simulink model "BCM2_4"  (R2021b)
settings: Solver=FixedStepDiscrete  StartTime=0.0  StopTime=1  FixedStep=0.001  RelTol=1e-3  EnableMultiTasking=on
InitFcn:
  | mbd_mpc_consistency_checks(bdroot(gcs));
model workspace (MAT data in the model file):
  CAN_rec : Simulink.Signal (value not decoded)
  CAN_transm_stat : Simulink.Signal (value not decoded)
  CAN_trm : Simulink.Signal (value not decoded)
  DITHER_CFB0 : Simulink.Parameter (value not decoded)
  DITHER_CFB1 : Simulink.Parameter (value not decoded)
  DITHER_CFB2 : Simulink.Parameter (value not decoded)
  DITHER_EN0 : Simulink.Parameter (value not decoded)
  DITHER_EN1 : Simulink.Parameter (value not decoded)
  DITHER_EN2 : Simulink.Parameter (value not decoded)
  DITHER_SIZE0 : Simulink.Parameter (value not decoded)
  DITHER_SIZE1 : Simulink.Parameter (value not decoded)
  DITHER_SIZE2 : Simulink.Parameter (value not decoded)
  DITHER_STEP0 : Simulink.Parameter (value not decoded)
  DITHER_STEP1 : Simulink.Parameter (value not decoded)
  DITHER_STEP2 : Simulink.Parameter (value not decoded)
  DITHER_SYNC0 : Simulink.Parameter (value not decoded)
  DITHER_SYNC1 : Simulink.Parameter (value not decoded)
  DITHER_SYNC2 : Simulink.Parameter (value not decoded)
  ECUMbut : Simulink.Signal (value not decoded)
  FAULTN : Simulink.Signal (value not decoded)
  FM0 : Simulink.Parameter (value not decoded)
  FM1 : Simulink.Parameter (value not decoded)
  FM2 : Simulink.Parameter (value not decoded)
  FME : Simulink.Parameter (value not decoded)
  Fsys_M : Simulink.Parameter (value not decoded)
  Fsys_N : Simulink.Parameter (value not decoded)
  Fsys_WDEN : Simulink.Parameter (value not decoded)
  Fsys_div : Simulink.Parameter (value not decoded)
  HL0 : Simulink.Parameter (value not decoded)
  HL1 : Simulink.Parameter (value not decoded)
  HL2 : Simulink.Parameter (value not decoded)
  IDIAG0 : Simulink.Parameter (value not decoded)
  IDIAG1 : Simulink.Parameter (value not decoded)
  IDIAG2 : Simulink.Parameter (value not decoded)
  Ivalve : Simulink.Signal (value not decoded)
  KI_index0 : Simulink.Parameter (value not decoded)
  KI_index1 : Simulink.Parameter (value not decoded)
  KI_index2 : Simulink.Parameter (value not decoded)
  PWM_Period0 : Simulink.Parameter (value not decoded)
  PWM_Period1 : Simulink.Parameter (value not decoded)
  PWM_Period2 : Simulink.Parameter (value not decoded)
  RESN : Simulink.Signal (value not decoded)
  SR0 : Simulink.Parameter (value not decoded)
  SR1 : Simulink.Parameter (value not decoded)
  SR2 : Simulink.Parameter (value not decoded)
  Vparam : Simulink.Signal (value not decoded)
  block_tle : Simulink.Signal (value not decoded)
  disp : Simulink.Signal (value not decoded)
  ee_adr : Simulink.Signal (value not decoded)
  ee_en_rd : Simulink.Signal (value not decoded)
  ee_en_wr : Simulink.Signal (value not decoded)
  ee_idle : Simulink.Signal (value not decoded)
  ee_read : Simulink.Signal (value not decoded)
  ee_recv : Simulink.Signal (value not decoded)
  ee_send : Simulink.Signal (value not decoded)
  in_stats : Simulink.Signal (value not decoded)
  inputs : Simulink.Signal (value not decoded)
  light : Simulink.Signal (value not decoded)
  out_drv : Simulink.Signal (value not decoded)
  out_drv_test : Simulink.Signal (value not decoded)
  out_test_en : Simulink.Signal (value not decoded)
  recv_spi2 : Simulink.Signal (value not decoded)
  ret : Simulink.Signal (value not decoded)
  spi_rcv_tle82453 : Simulink.Signal (value not decoded)
  tle82453_Ivlv : Simulink.Signal (value not decoded)
  tle82453_err : Simulink.Signal (value not decoded)
  tle82453_reset : Simulink.Signal (value not decoded)
  wtdg_CAN : Simulink.Signal (value not decoded)
symbols that are objects in the model workspace (value not decoded): CAN_rec, CAN_transm_stat, ECUMbut, inputs, Ivalve, out_drv_test, recv_spi2, ret, SR0, tle82453_Ivlv
undefined symbols (not defined in the file or in its folder): color, LQFP
libraries: simulink x68, mbd_mpc574x_ec_toolbox x50, canmsglib x42, hdlsllib x9, commutil2 x7, etargetslib x4
(part 5 of 6)

== system BCM2_4/CAN_Receive/RX_FIFO_Complete_Event2 buf 22-26/ID0X18FEEA2F buf = 23 ==
  Data : Inport
  Action Port : ActionPort  ActionPortLabel=case [ 419359279 ]:
  Constant : Constant  Value=0  OutDataTypeStr=uint16
  Data Store Write1 : DataStoreWrite  DataStoreName=wtdg_CAN  DataStoreElements=wtdg_CAN.w18FEEA2F  IndexOptions=Index vector (dialog)  Indices=1  OutputSizes=1
  Data Store Write2 : DataStoreWrite  DataStoreName=CAN_rec  DataStoreElements=CAN_rec.m18FEEA2F(:)  IndexOptions=Index vector (dialog)  Indices=1  OutputSizes=1
  wires:
  Constant/1 -> Data Store Write1/1
  Data/1 -> Data Store Write2/1

== system BCM2_4/CAN_Receive/RX_FIFO_Complete_Event2 buf 22-26/ID0X192 buf = 22 ==
  Data : Inport
  Action Port : ActionPort  ActionPortLabel=case [ 402 ]:
  CAN Pack1 : canmsglib/CAN Pack  CANdbFile=C:\Documents\Документация\J1939\j1939.dbc  MsgList=A1  MsgName=CANPACK  MsgIDType=Standard (11-bit identifier)  MsgIdentifier=hex2dec('192')  MsgLength=8  Remote=off  ApplyMinMax=off  BusOutput=off  SignalInfo={}
      settings: SourceProductBaseCode=ME,XP,VN  DataFormat=raw data
  CAN Unpack2 : canmsglib/CAN Unpack  MsgList=(none)  MsgName=Ecu_master_4  MsgIDType=Standard (11-bit identifier)  MsgIdentifier="hex2dec(\"192\")"  MsgLength=8  SignalInfo={ 'Butons', '0', '8', 'LE', 'signed', 'Standard', '0', '1', '0', '-Inf', 'Inf' }  IDPort=off  TimestampPort=off  ErrorPort=off  RemotePort=off  LengthPort=off  StatusPort=off  ApplyMinMax=off
      settings: SourceProductName=Simulink Real-Time
  Constant : Constant  Value=0  OutDataTypeStr=uint16
  Data Store Write : DataStoreWrite  DataStoreName=ECUMbut  DataStoreElements=ECUMbut.arr4(:)  IndexOptions=Index vector (dialog)  Indices=1  OutputSizes=1
  Data Store Write1 : DataStoreWrite  DataStoreName=wtdg_CAN  DataStoreElements=wtdg_CAN.id192  IndexOptions=Index vector (dialog)  Indices=1  OutputSizes=1
  Integer to Bit Converter : commutil2/Integer to Bit Converter  nbits=8  signedInputValues=Unsigned  bitOrder=LSB first  outDtype=boolean
  wires:
  Data/1 -> CAN Pack1/1
  CAN Unpack2/1 -> Integer to Bit Converter/1
  CAN Pack1/1 -> CAN Unpack2/1
  Constant/1 -> Data Store Write1/1
  Integer to Bit Converter/1 -> Data Store Write/1

== system BCM2_4/CAN_Receive/RX_FIFO_Complete_Event2 buf 22-26/ID0X195 buf = 22 ==
  Data : Inport
  Action Port : ActionPort  ActionPortLabel=case [ 405 ]:
  CAN Pack1 : canmsglib/CAN Pack  CANdbFile=C:\Documents\Документация\J1939\j1939.dbc  MsgList=A1  MsgName=CANPACK  MsgIDType=Standard (11-bit identifier)  MsgIdentifier=hex2dec('195')  MsgLength=8  Remote=off  ApplyMinMax=off  BusOutput=off  SignalInfo={}
      settings: SourceProductBaseCode=ME,XP,VN  DataFormat=raw data
  CAN Unpack1 : canmsglib/CAN Unpack  MsgList=(none)  MsgName=ecumaster_12  MsgIDType=Standard (11-bit identifier)  MsgIdentifier="hex2dec(\"195\")"  MsgLength=8  SignalInfo={ 'buttons', '0', '16', 'LE', 'unsigned', 'Standard', '0', '1', '0', '0', 'inf' }  IDPort=off  TimestampPort=off  ErrorPort=off  RemotePort=off  LengthPort=off  StatusPort=off  ApplyMinMax=off
      settings: SourceProductName=Simulink Real-Time
  Constant : Constant  Value=0  OutDataTypeStr=uint16
  Data Store Write : DataStoreWrite  DataStoreName=ECUMbut  DataStoreElements=ECUMbut.arr12(:)  IndexOptions=Index vector (dialog)  Indices=1  OutputSizes=1
  Data Store Write1 : DataStoreWrite  DataStoreName=wtdg_CAN  DataStoreElements=wtdg_CAN.id195  IndexOptions=Index vector (dialog)  Indices=1  OutputSizes=1
  Integer to Bit Converter : commutil2/Integer to Bit Converter  nbits=16  signedInputValues=Unsigned  bitOrder=LSB first  outDtype=boolean
  wires:
  CAN Pack1/1 -> CAN Unpack1/1
  Data/1 -> CAN Pack1/1
  CAN Unpack1/1 -> Integer to Bit Converter/1
  Integer to Bit Converter/1 -> Data Store Write/1
  Constant/1 -> Data Store Write1/1

== system BCM2_4/CAN_Receive/RX_FIFO_Complete_Event2 buf 22-26/reinit buf 22 ==
  Action Port : ActionPort  ActionPortLabel=case [ 22 ]:
  FCAN_Receive_ID_1xx : mbd_mpc574x_ec_toolbox/Communication Blocks/CAN Blocks/FCAN_Receive  can_instance=1  can_mode=Non-blocking  can_timeout_ms=0  can_mb_idx=22  can_extended_id=off  can_is_remote=off  can_id=100  can_msg_mask=FFFFFF00  show_adv_opts=off  can_use_rxfifo=off  can_fd_enable=off
      settings: SourceProductName=NXP Model-Based Design Toolbox for MPC57xx MCUs

== system BCM2_4/CAN_Receive/RX_FIFO_Complete_Event2 buf 22-26/reinit buf 23 ==
  Action Port : ActionPort  ActionPortLabel=case [ 23 ]:
  FCAN_Receive_ID_18Fxxxxx : mbd_mpc574x_ec_toolbox/Communication Blocks/CAN Blocks/FCAN_Receive  can_instance=1  can_mode=Non-blocking  can_timeout_ms=0  can_mb_idx=22  can_extended_id=on  can_is_remote=off  can_id=18F00000  can_msg_mask=FFF00000  show_adv_opts=off  can_use_rxfifo=off  can_fd_enable=off
      settings: SourceProductName=NXP Model-Based Design Toolbox for MPC57xx MCUs

== system BCM2_4/CAN_Receive/RX_FIFO_Complete_Event3 buf 44-48/ID0X192 buf = 15 ==
  Data : Inport
  Action Port : ActionPort
  CAN Pack1 : canmsglib/CAN Pack  CANdbFile=C:\Documents\Документация\J1939\j1939.dbc  MsgList=A1  MsgName=CANPACK  MsgIDType=Standard (11-bit identifier)  MsgIdentifier=hex2dec('192')  MsgLength=8  Remote=off  ApplyMinMax=off  BusOutput=off  SignalInfo={}
      settings: SourceProductBaseCode=ME,XP,VN  DataFormat=raw data
  CAN Unpack2 : canmsglib/CAN Unpack  MsgList=(none)  MsgName=Rear_modulator  MsgIDType=Standard (11-bit identifier)  MsgIdentifier="hex2dec(\"192\")"  MsgLength=8  SignalInfo={ 'Current_pressure', '48', '8', 'LE', 'unsigned', 'Standard', '0', '0.05', '0', '-Inf', 'Inf'; 'Select_pressure', '56', '8', 'LE', 'unsigned', 'Standard', '0', '0.05', '0', '-Inf', 'Inf' }  IDPort=off  TimestampPort=off  ErrorPort=off  RemotePort=off  LengthPort=off  StatusPort=off  ApplyMinMax=off
      settings: SourceProductName=Simulink Real-Time
  Constant : Constant  Value=0  OutDataTypeStr=uint16
  Data Store Write1 : DataStoreWrite  DataStoreName=wtdg_CAN  DataStoreElements=wtdg_CAN.id192  IndexOptions=Index vector (dialog)  Indices=1  OutputSizes=1
  Terminator : Terminator
  Terminator1 : Terminator
  wires:
  Constant/1 -> Data Store Write1/1
  CAN Pack1/1 -> CAN Unpack2/1
  CAN Unpack2/1 -> Terminator/1
  CAN Unpack2/2 -> Terminator1/1
  Data/1 -> CAN Pack1/1

== system BCM2_4/CAN_Receive/RX_FIFO_Complete_Event3 buf 44-48/ID0X195 buf = 15 ==
  Data : Inport
  Action Port : ActionPort
  CAN Pack1 : canmsglib/CAN Pack  CANdbFile=C:\Documents\Документация\J1939\j1939.dbc  MsgList=A1  MsgName=CANPACK  MsgIDType=Standard (11-bit identifier)  MsgIdentifier=hex2dec('195')  MsgLength=8  Remote=off  ApplyMinMax=off  BusOutput=off  SignalInfo={}
      settings: SourceProductBaseCode=ME,XP,VN  DataFormat=raw data
  CAN Unpack1 : canmsglib/CAN Unpack  MsgList=(none)  MsgName=ecumaster_12  MsgIDType=Standard (11-bit identifier)  MsgIdentifier="hex2dec(\"195\")"  MsgLength=8  SignalInfo={ 'buttons', '0', '16', 'LE', 'unsigned', 'Standard', '0', '1', '0', '0', 'inf' }  IDPort=off  TimestampPort=off  ErrorPort=off  RemotePort=off  LengthPort=off  StatusPort=off  ApplyMinMax=off
      settings: SourceProductName=Simulink Real-Time
  Constant : Constant  Value=0  OutDataTypeStr=uint16
  Data Store Write : DataStoreWrite  DataStoreName=ECUMbut  DataStoreElements=ECUMbut.arr12(:)  IndexOptions=Index vector (dialog)  Indices=1  OutputSizes=1
  Data Store Write1 : DataStoreWrite  DataStoreName=wtdg_CAN  DataStoreElements=wtdg_CAN.id195  IndexOptions=Index vector (dialog)  Indices=1  OutputSizes=1
  Integer to Bit Converter : commutil2/Integer to Bit Converter  nbits=16  signedInputValues=Unsigned  bitOrder=LSB first  outDtype=boolean
  wires:
  Constant/1 -> Data Store Write1/1
  Integer to Bit Converter/1 -> Data Store Write/1
  CAN Unpack1/1 -> Integer to Bit Converter/1
  Data/1 -> CAN Pack1/1
  CAN Pack1/1 -> CAN Unpack1/1

== system BCM2_4/CAN_Receive/RX_FIFO_Complete_Event3 buf 44-48/reinit buf 15 ==
  Action Port : ActionPort
  FCAN_Receive_ID_1xx : mbd_mpc574x_ec_toolbox/Communication Blocks/CAN Blocks/FCAN_Receive  can_instance=1  can_mode=Non-blocking  can_timeout_ms=0  can_mb_idx=15  can_extended_id=off  can_is_remote=off  can_id=100  can_msg_mask=FFFFFF00  show_adv_opts=off  can_use_rxfifo=off  can_fd_enable=off
      settings: SourceProductName=NXP Model-Based Design Toolbox for MPC57xx MCUs

== system BCM2_4/Drivers/Diagnostic1/Switch Case Action Subsystem ==
  In1 : Inport
  Action Port : ActionPort  ActionPortLabel=case [ 2 ]:
  Byte Unpack1 : etargetslib/Byte Unpack  dimensions={[1]}  datatypes={'uint32'}  byteAlign=4
  Constant : Constant  Value=0  OutDataTypeStr=uint8  SampleTime=-1
  Data Store Write : DataStoreWrite  DataStoreName=tle82453_err  IndexOptions=Index vector (dialog)  Indices=1  OutputSizes=1
  Mux : Mux  Inputs=2
  wires:
  Byte Unpack1/1 -> Data Store Write/1
  In1/1 -> Mux/2
  Mux/1 -> Byte Unpack1/1
  Constant/1 -> Mux/1

== system BCM2_4/Drivers/Diagnostic1/Switch Case Action Subsystem1 ==
  In1 : Inport
  Action Port : ActionPort  ActionPortLabel=case [ 64 ]:
  Add : Sum  Inputs=3
  Bit Shift1 : hdlsllib/Logic and Bit Operations/Bit Shift  mode=Shift Left Logical  N=8
  Bit Shift2 : hdlsllib/Logic and Bit Operations/Bit Shift  mode=Shift Right Logical  N=12
  Bit Shift3 : hdlsllib/Logic and Bit Operations/Bit Shift  mode=Shift Left Logical  N=16
  Bitwise AND : simulink/Logic and Bit Operations/Bitwise Operator  logicop=AND  UseBitMask=on  BitMask=bin2dec('000000000000111111111111')  BitMaskRealWorld=Stored Integer
  Data Store Write1 : DataStoreWrite  DataStoreName=tle82453_Ivlv  DataStoreElements=tle82453_Ivlv(1)  IndexOptions=Index vector (dialog)  Indices=1  OutputSizes=1
  Data Type Conversion : DataTypeConversion  OutDataTypeStr=uint32
  Data Type Conversion1 : DataTypeConversion  OutDataTypeStr=double
  Data Type Conversion2 : DataTypeConversion  OutDataTypeStr=double
  Data Type Conversion3 : DataTypeConversion  OutDataTypeStr=uint8
  Demux : Demux  Outputs=3
  Gain : Gain  Gain=150  OutDataTypeStr=double
  Multiply : Product  Inputs=*/  OutDataTypeStr=double
  wires:
  Bitwise AND/1 -> Data Type Conversion2/1
  Data Type Conversion2/1 -> Multiply/2
  Gain/1 -> Multiply/1
  Add/1 -> Bitwise AND/1, Bit Shift2/1
  Bit Shift3/1 -> Add/1
  Demux/3 -> Add/3
  Bit Shift2/1 -> Data Type Conversion1/1
  Data Type Conversion1/1 -> Gain/1
  Demux/1 -> Bit Shift3/1
  Bit Shift1/1 -> Add/2
  Demux/2 -> Bit Shift1/1
  Data Type Conversion/1 -> Demux/1
  In1/1 -> Data Type Conversion/1
  Data Type Conversion3/1 -> Data Store Write1/1
  Multiply/1 -> Data Type Conversion3/1

== system BCM2_4/Drivers/Diagnostic1/Switch Case Action Subsystem2 ==
  In1 : Inport
  Action Port : ActionPort  ActionPortLabel=case [ 65 ]:
  Add : Sum  Inputs=3
  Bit Shift1 : hdlsllib/Logic and Bit Operations/Bit Shift  mode=Shift Left Logical  N=8
  Bit Shift2 : hdlsllib/Logic and Bit Operations/Bit Shift  mode=Shift Right Logical  N=12
  Bit Shift3 : hdlsllib/Logic and Bit Operations/Bit Shift  mode=Shift Left Logical  N=16
  Bitwise AND : simulink/Logic and Bit Operations/Bitwise Operator  logicop=AND  UseBitMask=on  BitMask=bin2dec('000000000000111111111111')  BitMaskRealWorld=Stored Integer
  Data Store Write2 : DataStoreWrite  DataStoreName=tle82453_Ivlv  DataStoreElements=tle82453_Ivlv(2)  IndexOptions=Index vector (dialog)  Indices=1  OutputSizes=1
  Data Type Conversion : DataTypeConversion  OutDataTypeStr=uint32
  Data Type Conversion1 : DataTypeConversion  OutDataTypeStr=double
  Data Type Conversion2 : DataTypeConversion  OutDataTypeStr=double
  Data Type Conversion3 : DataTypeConversion  OutDataTypeStr=uint8
  Demux : Demux  Outputs=3
  Gain : Gain  Gain=150  OutDataTypeStr=double
  Multiply : Product  Inputs=*/  OutDataTypeStr=double
  wires:
  Bit Shift2/1 -> Data Type Conversion1/1
  Demux/2 -> Bit Shift1/1
  Data Type Conversion/1 -> Demux/1
  Bit Shift1/1 -> Add/2
  Demux/3 -> Add/3
  Add/1 -> Bitwise AND/1, Bit Shift2/1
  Bit Shift3/1 -> Add/1
  Demux/1 -> Bit Shift3/1
  In1/1 -> Data Type Conversion/1
  Bitwise AND/1 -> Data Type Conversion2/1
  Gain/1 -> Multiply/1
  Data Type Conversion1/1 -> Gain/1
  Data Type Conversion2/1 -> Multiply/2
  Data Type Conversion3/1 -> Data Store Write2/1
  Multiply/1 -> Data Type Conversion3/1

== system BCM2_4/Drivers/Diagnostic1/Switch Case Action Subsystem3 ==
  In1 : Inport
  Action Port : ActionPort  ActionPortLabel=case [ 66 ]:
  Add : Sum  Inputs=3
  Bit Shift1 : hdlsllib/Logic and Bit Operations/Bit Shift  mode=Shift Left Logical  N=8
  Bit Shift2 : hdlsllib/Logic and Bit Operations/Bit Shift  mode=Shift Right Logical  N=12
  Bit Shift3 : hdlsllib/Logic and Bit Operations/Bit Shift  mode=Shift Left Logical  N=16
  Bitwise AND : simulink/Logic and Bit Operations/Bitwise Operator  logicop=AND  UseBitMask=on  BitMask=bin2dec('000000000000111111111111')  BitMaskRealWorld=Stored Integer
  Data Store Write3 : DataStoreWrite  DataStoreName=tle82453_Ivlv  DataStoreElements=tle82453_Ivlv(3)  IndexOptions=Index vector (dialog)  Indices=1  OutputSizes=1
  Data Type Conversion : DataTypeConversion  OutDataTypeStr=uint32
  Data Type Conversion1 : DataTypeConversion  OutDataTypeStr=double
  Data Type Conversion2 : DataTypeConversion  OutDataTypeStr=double
  Data Type Conversion3 : DataTypeConversion  OutDataTypeStr=uint8
  Demux : Demux  Outputs=3
  Gain : Gain  Gain=150  OutDataTypeStr=double
  Multiply : Product  Inputs=*/  OutDataTypeStr=double
  wires:
  In1/1 -> Data Type Conversion/1
  Bitwise AND/1 -> Data Type Conversion2/1
  Data Type Conversion2/1 -> Multiply/2
  Gain/1 -> Multiply/1
  Add/1 -> Bitwise AND/1, Bit Shift2/1
  Bit Shift3/1 -> Add/1
  Demux/3 -> Add/3
  Bit Shift2/1 -> Data Type Conversion1/1
  Data Type Conversion1/1 -> Gain/1
  Demux/1 -> Bit Shift3/1
  Bit Shift1/1 -> Add/2
  Demux/2 -> Bit Shift1/1
  Data Type Conversion/1 -> Demux/1
  Data Type Conversion3/1 -> Data Store Write3/1
  Multiply/1 -> Data Type Conversion3/1

== system BCM2_4/Drivers/input status/Switch Case Action Subsystem ==
  Action Port : ActionPort  ActionPortLabel=case [ 62 ]:
  Byte Unpack : etargetslib/Byte Unpack  dimensions={[1]}  datatypes={'uint32'}  byteAlign=4
  Data Store Read1 : DataStoreRead  DataStoreName=recv_spi2  DataStoreElements=recv_spi2(1:4)  IndexOptions=Index vector (dialog)  Indices=1  OutputSizes=1
  Data Store Write1 : DataStoreWrite  DataStoreName=inputs  DataStoreElements=inputs(1:22)  IndexOptions=Index vector (dialog)  Indices=1  OutputSizes=1
  Integer to Bit Converter1 : commutil2/Integer to Bit Converter  nbits=32  signedInputValues=Unsigned  bitOrder=LSB first  outDtype=boolean
  Selector2 : Selector  InputPortWidth=32  IndexOptions=Index vector (dialog)  Indices=[1:22]  OutputSizes=1
  wires:
  Selector2/1 -> Data Store Write1/1
  Integer to Bit Converter1/1 -> Selector2/1
  Data Store Read1/1 -> Byte Unpack/1
  Byte Unpack/1 -> Integer to Bit Converter1/1

== system BCM2_4/Drivers/input status/Switch Case Action Subsystem1 ==
  Action Port : ActionPort  ActionPortLabel=default:

== system BCM2_4/Drivers/input status/Switch Case Action Subsystem2 ==
  Action Port : ActionPort  ActionPortLabel=case [ 62 ]:
  Byte Unpack : etargetslib/Byte Unpack  dimensions={[1]}  datatypes={'uint32'}  byteAlign=4
  Data Store Read : DataStoreRead  DataStoreName=recv_spi2  DataStoreElements=recv_spi2(5:8)  IndexOptions=Index vector (dialog)  Indices=1  OutputSizes=1
  Data Store Write : DataStoreWrite  DataStoreName=inputs  DataStoreElements=inputs(23:44)  IndexOptions=Index vector (dialog)  Indices=1  OutputSizes=1
  Integer to Bit Converter1 : commutil2/Integer to Bit Converter  nbits=32  signedInputValues=Unsigned  bitOrder=LSB first  outDtype=boolean
  Selector2 : Selector  InputPortWidth=32  IndexOptions=Index vector (dialog)  Indices=[1:22]  OutputSizes=1
  wires:
  Byte Unpack/1 -> Integer to Bit Converter1/1
  Selector2/1 -> Data Store Write/1
  Integer to Bit Converter1/1 -> Selector2/1
  Data Store Read/1 -> Byte Unpack/1

== system BCM2_4/Drivers/input status/Switch Case Action Subsystem3 ==
  Action Port : ActionPort  ActionPortLabel=default:

== system BCM2_4/Init System/Начальная иницилизация/Init filters CAN ==
  FCAN_Receive_ID_0CFxxxxx : mbd_mpc574x_ec_toolbox/Communication Blocks/CAN Blocks/FCAN_Receive  can_instance=0  can_mode=Non-blocking  can_timeout_ms=0  can_mb_idx=0  can_extended_id=on  can_is_remote=off  can_id=0CF00000  can_msg_mask=FFF00000  show_adv_opts=off  can_use_rxfifo=off  can_fd_enable=off
      settings: SourceProductName=NXP Model-Based Design Toolbox for MPC57xx MCUs
  FCAN_Receive_ID_1811xxxxx : mbd_mpc574x_ec_toolbox/Communication Blocks/CAN Blocks/FCAN_Receive  can_instance=0  can_mode=Non-blocking  can_timeout_ms=0  can_mb_idx=2  can_extended_id=on  can_is_remote=off  can_id=18110000  can_msg_mask=FFFF0000  show_adv_opts=off  can_use_rxfifo=off  can_fd_enable=off
      settings: SourceProductName=NXP Model-Based Design Toolbox for MPC57xx MCUs
  FCAN_Receive_ID_18Fxxxxx : mbd_mpc574x_ec_toolbox/Communication Blocks/CAN Blocks/FCAN_Receive  can_instance=0  can_mode=Non-blocking  can_timeout_ms=0  can_mb_idx=1  can_extended_id=on  can_is_remote=off  can_id=18F00000  can_msg_mask=FFF00000  show_adv_opts=off  can_use_rxfifo=off  can_fd_enable=off
      settings: SourceProductName=NXP Model-Based Design Toolbox for MPC57xx MCUs
  FCAN_Receive_ID_18Fxxxxx1 : mbd_mpc574x_ec_toolbox/Communication Blocks/CAN Blocks/FCAN_Receive  can_instance=1  can_mode=Non-blocking  can_timeout_ms=0  can_mb_idx=22  can_extended_id=on  can_is_remote=off  can_id=18F00000  can_msg_mask=FFF00000  show_adv_opts=off  can_use_rxfifo=off  can_fd_enable=off
      settings: SourceProductName=NXP Model-Based Design Toolbox for MPC57xx MCUs
  FCAN_Receive_ID_1FEEF888 : mbd_mpc574x_ec_toolbox/Communication Blocks/CAN Blocks/FCAN_Receive  can_instance=0  can_mode=Non-blocking  can_timeout_ms=0  can_mb_idx=3  can_extended_id=on  can_is_remote=off  can_id=1FEEF888  can_msg_mask=FFFFFFFF  show_adv_opts=off  can_use_rxfifo=off  can_fd_enable=off
      settings: SourceProductName=NXP Model-Based Design Toolbox for MPC57xx MCUs
  FCAN_Receive_ID_1xx : mbd_mpc574x_ec_toolbox/Communication Blocks/CAN Blocks/FCAN_Receive  can_instance=1  can_mode=Non-blocking  can_timeout_ms=0  can_mb_idx=22  can_extended_id=off  can_is_remote=off  can_id=100  can_msg_mask=FFFFFF00  show_adv_opts=off  can_use_rxfifo=off  can_fd_enable=off
      settings: SourceProductName=NXP Model-Based Design Toolbox for MPC57xx MCUs

== system BCM2_4/Степы ретардера/страницы механика+/Subsystem ==
  Enable : EnablePort
  Add : Sum
  Constant : Constant  OutDataTypeStr=uint8
  Data Store Read : DataStoreRead  DataStoreName=ret  DataStoreElements=ret.step  IndexOptions=Index vector (dialog)  Indices=1  OutputSizes=1
  Data Store Write : DataStoreWrite  DataStoreName=ret  DataStoreElements=ret.step  IndexOptions=Index vector (dialog)  Indices=1  OutputSizes=1
  wires:
  Constant/1 -> Add/2
  Data Store Read/1 -> Add/1
  Add/1 -> Data Store Write/1

== system BCM2_4/Степы ретардера/страницы механика+/Subsystem1 ==
  Enable : EnablePort
  Add : Sum
  Constant : Constant  OutDataTypeStr=uint8
  Data Store Read : DataStoreRead  DataStoreName=ret  DataStoreElements=ret.step_brk  IndexOptions=Index vector (dialog)  Indices=1  OutputSizes=1
  Data Store Write : DataStoreWrite  DataStoreName=ret  DataStoreElements=ret.step_brk  IndexOptions=Index vector (dialog)  Indices=1  OutputSizes=1
  wires:
  Add/1 -> Data Store Write/1
  Data Store Read/1 -> Add/1
  Constant/1 -> Add/2

== system BCM2_4/Степы ретардера/страницы механика-/Subsystem ==
  Enable : EnablePort
  Add : Sum  Inputs=+-
  Constant : Constant  OutDataTypeStr=uint8
  Data Store Read : DataStoreRead  DataStoreName=ret  DataStoreElements=ret.step  IndexOptions=Index vector (dialog)  Indices=1  OutputSizes=1
  Data Store Write : DataStoreWrite  DataStoreName=ret  DataStoreElements=ret.step  IndexOptions=Index vector (dialog)  Indices=1  OutputSizes=1
  wires:
  Add/1 -> Data Store Write/1
  Data Store Read/1 -> Add/1
  Constant/1 -> Add/2

== system BCM2_4/Топливные баки/Enabled Subsystem/Subsystem ==
  Enable : EnablePort
  Add : Sum  Inputs=+-
  Add1 : Sum
  Constant : Constant  Value=0.8
  Constant1 : Constant  Value=0.8
  Data Store Read : DataStoreRead  DataStoreName=tank1  SampleTime=1  IndexOptions=Index vector (dialog)  Indices=1  OutputSizes=1
  Data Store Read1 : DataStoreRead  DataStoreName=tank3  SampleTime=1  IndexOptions=Index vector (dialog)  Indices=1  OutputSizes=1
  Data Store Write : DataStoreWrite  DataStoreName=tank1  IndexOptions=Index vector (dialog)  Indices=1  OutputSizes=1
  Data Store Write1 : DataStoreWrite  DataStoreName=tank3  IndexOptions=Index vector (dialog)  Indices=1  OutputSizes=1
  wires:
  Constant/1 -> Add/2
  Add/1 -> Data Store Write/1
  Data Store Read/1 -> Add/1
  Data Store Read1/1 -> Add1/1
  Add1/1 -> Data Store Write1/1
  Constant1/1 -> Add1/2

== system BCM2_4/Топливные баки/Enabled Subsystem1/Subsystem ==
  Enable : EnablePort
  Add : Sum  Inputs=+-
  Add1 : Sum
  Constant : Constant  Value=0.8
  Constant1 : Constant  Value=0.8
  Data Store Read : DataStoreRead  DataStoreName=tank2  SampleTime=1  IndexOptions=Index vector (dialog)  Indices=1  OutputSizes=1
  Data Store Read1 : DataStoreRead  DataStoreName=tank3  SampleTime=1  IndexOptions=Index vector (dialog)  Indices=1  OutputSizes=1
  Data Store Write : DataStoreWrite  DataStoreName=tank2  IndexOptions=Index vector (dialog)  Indices=1  OutputSizes=1
  Data Store Write1 : DataStoreWrite  DataStoreName=tank3  IndexOptions=Index vector (dialog)  Indices=1  OutputSizes=1
  wires:
  Constant1/1 -> Add1/2
  Add1/1 -> Data Store Write1/1
  Data Store Read1/1 -> Add1/1
  Data Store Read/1 -> Add/1
  Add/1 -> Data Store Write/1
  Constant/1 -> Add/2

== system BCM2_4/Управление с клавиатуры ECUMASTER/Переключение таблиц ДВС/сброс на ноль ==
  Enable : EnablePort
  Constant : Constant  Value=0  OutDataTypeStr=uint8
  Data Store Write1 : DataStoreWrite  DataStoreName=ECUMbut  DataStoreElements=ECUMbut.cnt(2)  IndexOptions=Index vector (dialog)  Indices=1  OutputSizes=1
  wires:
  Constant/1 -> Data Store Write1/1

== system BCM2_4/Управление с клавиатуры ECUMASTER/Управление габаритами и ближним2/сброс на ноль ==
  Enable : EnablePort
  Constant : Constant  Value=0  OutDataTypeStr=uint8
  Data Store Write1 : DataStoreWrite  DataStoreName=ECUMbut  DataStoreElements=ECUMbut.cnt(1)  IndexOptions=Index vector (dialog)  Indices=1  OutputSizes=1
  wires:
  Constant/1 -> Data Store Write1/1

== system BCM2_4/управление страницами и яркостью мониторов/страницы механика+/Subsystem ==
  Enable : EnablePort
  Add : Sum
  Constant : Constant  OutDataTypeStr=uint8
  Data Store Read : DataStoreRead  DataStoreName=disp  DataStoreElements=disp.meh_page  IndexOptions=Index vector (dialog)  Indices=1  OutputSizes=1
  Data Store Write : DataStoreWrite  DataStoreName=disp  DataStoreElements=disp.meh_page  IndexOptions=Index vector (dialog)  Indices=1  OutputSizes=1
  wires:
  Constant/1 -> Add/2
  Data Store Read/1 -> Add/1
  Add/1 -> Data Store Write/1

== system BCM2_4/управление страницами и яркостью мониторов/страницы механика-/Subsystem ==
  Enable : EnablePort
  Add : Sum  Inputs=+-
  Constant : Constant  OutDataTypeStr=uint8
  Data Store Read : DataStoreRead  DataStoreName=disp  DataStoreElements=disp.meh_page  IndexOptions=Index vector (dialog)  Indices=1  OutputSizes=1
  Data Store Write : DataStoreWrite  DataStoreName=disp  DataStoreElements=disp.meh_page  IndexOptions=Index vector (dialog)  Indices=1  OutputSizes=1
  wires:
  Add/1 -> Data Store Write/1
  Data Store Read/1 -> Add/1
  Constant/1 -> Add/2

== system BCM2_4/управление страницами и яркостью мониторов/страницы пилота+/Subsystem ==
  Enable : EnablePort
  Add : Sum
  Constant : Constant  OutDataTypeStr=uint8
  Data Store Read : DataStoreRead  DataStoreName=disp  DataStoreElements=disp.pilot_page  IndexOptions=Index vector (dialog)  Indices=1  OutputSizes=1
  Data Store Write : DataStoreWrite  DataStoreName=disp  DataStoreElements=disp.pilot_page  IndexOptions=Index vector (dialog)  Indices=1  OutputSizes=1
  wires:
  Add/1 -> Data Store Write/1
  Data Store Read/1 -> Add/1
  Constant/1 -> Add/2

== system BCM2_4/управление страницами и яркостью мониторов/страницы пилота-/Subsystem ==
  Enable : EnablePort
  Add : Sum  Inputs=+-
  Constant : Constant  OutDataTypeStr=uint8
  Data Store Read : DataStoreRead  DataStoreName=disp  DataStoreElements=disp.pilot_page  IndexOptions=Index vector (dialog)  Indices=1  OutputSizes=1
  Data Store Write : DataStoreWrite  DataStoreName=disp  DataStoreElements=disp.pilot_page  IndexOptions=Index vector (dialog)  Indices=1  OutputSizes=1
  wires:
  Constant/1 -> Add/2
  Data Store Read/1 -> Add/1
  Add/1 -> Data Store Write/1

== stateflow chart BCM2_4/Drivers/Driver TLE82453-3 ==
  settings: updateMethod=DISCRETE  sampleTime=0.001
  state Start
    state Init_Vars1
      CLK_DIVIDER = 0x83000000
      CLK_DIVIDER =bitor(CLK_DIVIDER , bitshift(Fsys_WDEN, 12))
      CLK_DIVIDER =bitor(CLK_DIVIDER , bitshift(Fsys_M, 6))
      CLK_DIVIDER =bitor(CLK_DIVIDER , bitshift(Fsys_N, 2))
      CLK_DIVIDER =bitor(CLK_DIVIDER , Fsys_div)
      %-------------------------------------------------------------------------------------
      PWM_PERIOD0 = 0xA8000000
      PWM_PERIOD0 =bitor(PWM_PERIOD0 , bitshift(0, 24))
      PWM_PERIOD0 =bitor(PWM_PERIOD0 , bitshift(KI_index0, 20))
      PWM_PERIOD0 =bitor(PWM_PERIOD0 , PWM_Period0)
      PWM_PERIOD1 = 0xA8000000
      PWM_PERIOD1 =bitor(PWM_PERIOD1 , bitshift(1, 24))
      PWM_PERIOD1 =bitor(PWM_PERIOD1 , bitshift(KI_index1, 20))
      PWM_PERIOD1 =bitor(PWM_PERIOD1 , PWM_Period1)
      PWM_PERIOD2 = 0xA8000000
      PWM_PERIOD2 =bitor(PWM_PERIOD2 , bitshift(2, 24))
      PWM_PERIOD2 =bitor(PWM_PERIOD2 , bitshift(KI_index2, 20))
      PWM_PERIOD2 =bitor(PWM_PERIOD2 , PWM_Period2)
      %--------------------------------------------------------------------------------------
      DITHER0 = 0x98000000
      DITHER0 =bitor(DITHER0 , bitshift(0, 24))
      DITHER0 =bitor(DITHER0 , bitshift(DITHER_EN0, 23))
      DITHER0 =bitor(DITHER0 , bitshift(DITHER_SYNC0, 22))
      DITHER0 =bitor(DITHER0 , bitshift(DITHER_CFB0, 21))
      DITHER0 =bitor(DITHER0 , bitshift(DITHER_STEP0, 10))
      DITHER0 =bitor(DITHER0 , DITHER_SIZE0)
      DITHER1 = 0x98000000
      DITHER1 =bitor(DITHER1 , bitshift(1, 24))
      DITHER1 =bitor(DITHER1 , bitshift(DITHER_EN1, 23))
      DITHER1 =bitor(DITHER1 , bitshift(DITHER_SYNC1, 22))
      DITHER1 =bitor(DITHER1 , bitshift(DITHER_CFB1, 21))
      DITHER1 =bitor(DITHER1 , bitshift(DITHER_STEP1, 10))
      DITHER1 =bitor(DITHER1 , DITHER_SIZE1)
      DITHER2 = 0x98000000
      DITHER2 =bitor(DITHER2 , bitshift(1, 24))
      DITHER2 =bitor(DITHER2 , bitshift(DITHER_EN2, 23))
      DITHER2 =bitor(DITHER2 , bitshift(DITHER_SYNC2, 22))
      DITHER2 =bitor(DITHER2 , bitshift(DITHER_CFB2, 21))
      DITHER2 =bitor(DITHER2 , bitshift(DITHER_STEP2, 10))
      DITHER2 =bitor(DITHER2 , DITHER_SIZE2)
      %-------------------------------------------------------------------------------------
      CONF_REGISTER = 0x81000000
      CONF_REGISTER =bitor(CONF_REGISTER , bitshift((IDIAG2 - 1), 15))
      CONF_REGISTER =bitor(CONF_REGISTER , bitshift((IDIAG1 - 1), 14))
      CONF_REGISTER =bitor(CONF_REGISTER , bitshift((IDIAG0 - 1), 13))
      CONF_REGISTER =bitor(CONF_REGISTER , bitshift((SR2 - 1), 11))
      CONF_REGISTER =bitor(CONF_REGISTER , bitshift((SR1 - 1), 9))
      CONF_REGISTER =bitor(CONF_REGISTER , bitshift((SR0 - 1), 7))
      CONF_REGISTER =bitor(CONF_REGISTER , bitshift((FME - 1), 6))
      CONF_REGISTER =bitor(CONF_REGISTER , bitshift((FM2 - 1), 5))
      CONF_REGISTER =bitor(CONF_REGISTER , bitshift((FM1 - 1), 4))
      CONF_REGISTER =bitor(CONF_REGISTER , bitshift((FM0 - 1), 3))
      CONF_REGISTER =bitor(CONF_REGISTER , bitshift((HL2 - 1), 2))
      CONF_REGISTER =bitor(CONF_REGISTER , bitshift((HL1 - 1), 1))
      CONF_REGISTER =bitor(CONF_REGISTER , (HL0 - 1))
      %init_reg = typecast(swapbytes(CLK_DIVIDER), 'uint8')
      init_reg = typecast(CLK_DIVIDER, 'uint8')
      pwm_reg0 = typecast(PWM_PERIOD0, 'uint8')
      pwm_reg1 = typecast(PWM_PERIOD1, 'uint8')
      pwm_reg2 = typecast(PWM_PERIOD2, 'uint8')
      dith_reg0 = typecast(DITHER0, 'uint8')
      dith_reg1 = typecast(DITHER1, 'uint8')
      dith_reg2 = typecast(DITHER2, 'uint8')
      conf_reg = typecast(CONF_REGISTER, 'uint8')
    state init1
      RESN = false
    state init
      RESN = true
    state out_data
      out = init_reg
      send_spi
    state send
      out2 =  [0X30, bitand(out_drv,255,'uint16')]
      send_spi2
    state send1
      out2 = [0X3F, bitshift(out_drv,-8)]
      send_spi2
    (default) -> Init_Vars1
    Init_Vars1 -> init1
    init1 -> init
    init -> out_data
    send1 -> out_data
    out_data -> send
    send -> send1
  state Work_cycle
    state Setpoint
      out=SP
      res=setpoint(ch+1)*1.364
      IH_temp = bitshift(res,-8,'uint16')
      IL_temp = bitand(res,255,'uint16')
      out(1)=bitor(SP(1), ch)
      out(3)=IH_temp
      out(4)=IL_temp
      ch=ch+1
      send_spi
    state Feedback
      out=FB
      out(1)=bitor(FB(1), ch)
      ch=ch+1
      send_spi
    state Diag
      out=DIAG
      send_spi
    state send2
      out2 = [0X30, bitand(out_drv,255,'uint16')]
      send_spi2
    state send3
      out2 = [0X3F, bitshift(out_drv,-8)]
      send_spi2
    (default) -> Setpoint
    send3 -> Setpoint
    Setpoint -> Feedback : [ch>2]{ch=0}
    Feedback -> Diag : [ch>2]{ch=0}
    Diag -> send2
    send2 -> send3
  state CONFIG1
    state Autozero
      out=Autozero
      out(1) = bitor(Autozero(1),ch)
      ch = ch +1
      send_spi
    state Config
      out=conf_reg;
      send_spi
    state THRESHOLD
      out=ITO
      out(1) = bitor(ITO(1),ch)
      ch=ch+1
      send_spi
    state LIMIT
      out=IL
      out(1) = bitor(IL(1),ch)
      ch=ch+1
      send_spi
    (default) -> Autozero
    Autozero -> Config : [ch>2]{ch=0}
    Config -> THRESHOLD
    THRESHOLD -> LIMIT : [ch>2]{ch=0}
  state PWM_period1
    out=pwm_reg0
    send_spi
  state PWM_period2
    out=pwm_reg1
    send_spi
  state PWM_period3
    out=pwm_reg2
    send_spi
  state Dither1
    out=dith_reg0
    send_spi
  state Dither2
    out=dith_reg1
    send_spi
  state Dither3
    out=dith_reg2
    send_spi
  (default) -> Start
  Work_cycle -> Start : [FAULTN==false || RESET >0]
  Start -> CONFIG1 : [FAULTN==true]{ch=0;}
  CONFIG1 -> Start [order 1] : [FAULTN==false || RESET >0]
  CONFIG1 -> PWM_period1 [order 2] : [ch>2]{ch=0}
  PWM_period1 -> PWM_period2
  PWM_period2 -> PWM_period3
  Dither3 -> Work_cycle
  PWM_period3 -> Dither1
  Dither1 -> Dither2
  Dither2 -> Dither3
  data: Fsys_div parameter uint32 size=1; Fsys_N parameter uint32 size=1; Fsys_M parameter uint32 size=1; Fsys_WDEN parameter uint32 size=1; PWM_Period1 parameter uint32 size=1; PWM_Period2 parameter uint32 size=1; KI_index0 parameter uint32 size=1; KI_index1 parameter uint32 size=1; KI_index2 parameter uint32 size=1; PWM_PERIOD1 local uint32 size=1; PWM_PERIOD2 local uint32 size=1; PWM_Period0 parameter uint32 size=1; PWM_PERIOD0 local uint32 size=1; DITHER_EN0 parameter uint32 size=1; DITHER_EN1 parameter uint32 size=1; DITHER_EN2 parameter uint32 size=1; DITHER_SYNC0 parameter uint32 size=1; DITHER_SYNC1 parameter uint32 size=1; DITHER_SYNC2 parameter uint32 size=1; DITHER_CFB0 parameter uint32 size=1; DITHER_CFB1 parameter uint32 size=1; DITHER_CFB2 parameter uint32 size=1; DITHER_STEP0 parameter uint32 size=1; DITHER_STEP1 parameter uint32 size=1; DITHER_STEP2 parameter uint32 size=1; DITHER_SIZE0 parameter uint32 size=1; DITHER_SIZE1 parameter uint32 size=1; DITHER_SIZE2 parameter uint32 size=1; DITHER1 local uint32 size=1; DITHER2 local uint32 size=1; CLK_DIVIDER local uint32 size=1; ITO local uint8 size=[1 4] =[0XB0 0X00 0X00 0X00]; Autozero constant uint8 size=[1 4] =[0XB8 0X80 0X00 0X00]; SP local uint8 size=[1 4] =[0X90 0XC0 0X00 0X00]; FB local uint8 size=[1 4] =[0X40 0X00 0X00 0X00]; DIAG local uint8 size=[1 4] =[0X02 0X00 0X00 0X00]; IL local uint8 size=[1 4] =[0XA0 0XC8 0X0C 0X80]; IDIAG0 parameter uint32 size=1; CONF_REGISTER local uint32 size=1; SR0 parameter uint32 size=1; FME parameter uint32 size=1; FM0 parameter uint32 size=1; HL0 parameter uint32 size=1; SR1 parameter uint32 size=1; SR2 parameter uint32 size=1; FM1 parameter uint32 size=1; FM2 parameter uint32 size=1; IDIAG1 parameter uint32 size=1; IDIAG2 parameter uint32 size=1; HL1 parameter uint32 size=1; HL2 parameter uint32 size=1; DITHER0 local uint32 size=1; init_reg local uint8 size=[1 4]; pwm_reg0 local uint8 size=[1 4]; dith_reg0 local uint8 size=[1 4]; conf_reg local uint8 size=[1 4]; pwm_reg1 local uint8 size=[1 4]; pwm_reg2 local uint8 size=[1 4]; dith_reg1 local uint8 size=[1 4]; dith_reg2 local uint8 size=[1 4]; ch local uint8 size=1; FAULTN input boolean; RESET input boolean size=1; RESN output boolean size=1; setpoint input uint16 size=[1 3]; IH_temp local; IL_temp local; res local; out output uint8 size=[1 4]; out2 output uint8 size=[1 2]; out_drv input uint16 size=1
  events: send_spi output FUNCTION_CALL_EVENT; send_spi2 output FUNCTION_CALL_EVENT

== stateflow chart BCM2_4/CAN1 Transmit buf 27-43/Цвет клавиатуры 4 buf = 30/Цвет клавиатуры buf = 30/Chart ==
  (default) -> (junction 58)
  (junction 58) -> (junction 46) : {temp=0;}
  (junction 46) -> (junction 48) : {i=0;}
  (junction 48) -> (junction 57) [order 2] : {out[0] = (temp & 255);
      |  out[1] = (temp>>8) & 255;
      |  out[2] = (temp>>16)  & 255;
      |  out[3] = (temp>>24)  & 255;}
  (junction 48) -> (junction 47) [order 1] : [i<4]
  (junction 50) -> (junction 48)
  (junction 47) -> (junction 49) : {temp = temp | (input[i] & 1) << (0+i);
      | temp = temp | ((input[i] & 2)>>1) << (8 + i);
      | temp = temp | ((input[i] & 4)>>2) << (16 + i);}
  (junction 49) -> (junction 50) : {i++;}
  data: i local uint8 size=1 =uint8(0); input input uint8 size=4; temp local double size=1; out output uint8 size=8

== stateflow chart BCM2_4/Drivers/EEPROM DRIVER1 ==
  state start
  state Delay4
  state read_ee
    temp_adress = uint16(adress*2)
    hi_temp = bitshift(temp_adress,-8,'uint16')
    low_temp = bitand(temp_adress,255,'uint16')
    out_data(1) = 3
    out_data(2) = hi_temp
    out_data(3) = low_temp
    send_spi
  state cmd_write
    wr_cmd
    temp_adress = uint16(adress*2)
  state wite_flag
    flag_idle = false
  state write_ee
    hi_temp = bitshift(temp_adress,-8,'uint16')
    low_temp = bitand(temp_adress,255,'uint16')
    out_data(1) = 2
    out_data(2) = hi_temp
    out_data(3) = low_temp
    hi_temp = bitshift(in_data,-8,'uint16')
    low_temp = bitand(in_data,255,'uint16')
    out_data(4) = hi_temp
    out_data(5) = low_temp
    send_spi
  state memcpy
    mem_rd
  state Delay
  state Delay2
  state read_ee1
    out_data(1) = 3
    out_data(2) = hi_temp
    out_data(3) = low_temp
    send_spi
  state Delay3
  (default) -> start
  start -> cmd_write [order 1] : [wr_en]{flag_idle = true}
  start -> read_ee [order 2] : [rd_en]{flag_idle = true}
  Delay4 -> start
  wite_flag -> Delay4 : [~wr_en && ~rd_en]
  cmd_write -> write_ee
  memcpy -> wite_flag
  Delay -> read_ee
  read_ee -> Delay2
  Delay3 -> memcpy
  write_ee -> Delay
  Delay2 -> read_ee1
  read_ee1 -> Delay3
  data: hi_temp local uint16; low_temp local uint16; adress input uint8; wr_en input boolean; in_data input uint16; out_data output uint8 size=[1 5]; rd_en input boolean; temp_adress local uint16; flag_idle output boolean
  events: wr_cmd output FUNCTION_CALL_EVENT; send_spi output FUNCTION_CALL_EVENT; mem_rd output FUNCTION_CALL_EVENT

== stateflow chart BCM2_4/Степы ретардера/Степы ретардера ==
  settings: updateMethod=DISCRETE  sampleTime=0.01
  state Page_mehanic [parallel]
    settings: executionOrder=2
    state idle
    state start
    state page3
      en: Step_ret = 3
      du:
    state page4
      en: Step_ret = 4
      du:
    state page1
      en: Step_ret = 1
    state page2
      en: Step_ret = 2
      du:
    state page5
      en: Step_ret = 5
      du:
    state page6
      en: Step_ret = 6
      du:
    state ee_write
      en:send(ee_wr,EEPROM_WR)
    state ee_write1
      en:send(ee_wr,EEPROM_WR)
    state ee_write2
      en:send(ee_wr,EEPROM_WR)
    state ee_write3
      en:send(ee_wr,EEPROM_WR)
    state ee_write4
      en:send(ee_wr,EEPROM_WR)
    state ee_write5
      en:send(ee_wr,EEPROM_WR)
    (default) -> Page_mehanic.idle
    Page_mehanic.idle -> start : [ee_rd_ok]
    start -> page1 [order 6] : {Step_ret = 1}
    start -> page2 [order 1] : [Step_ret == 2]
    start -> page3 [order 3] : [Step_ret == 3]
    start -> page4 [order 4] : [Step_ret == 4]
    start -> page5 [order 5] : [Step_ret == 5]
    start -> page6 [order 2] : [Step_ret == 6]
    page3 -> page4 [order 1] : step_P{stat_wr = true}
    page2 -> page3 [order 1] : step_P{stat_wr = true}
    page4 -> page5 [order 1] : step_P{stat_wr = true}
    page1 -> page2 [order 2] : step_P{stat_wr = true}
    page5 -> page6 [order 2] : step_P{stat_wr = true}
    page4 -> page3 [order 3] : step_M{stat_wr = true}
    page3 -> page2 [order 3] : step_M{stat_wr = true}
    page5 -> page4 [order 1] : step_M{stat_wr = true}
    page2 -> page1 [order 3] : step_M{stat_wr = true}
    page6 -> page5 [order 2] : step_M{stat_wr = true}
    page2 -> ee_write1 [order 2] : [stat_wr && in(EEPROM_WR.idle)]
    ee_write1 -> page2 : {stat_wr = false}
    page1 -> ee_write [order 1] : [stat_wr && in(EEPROM_WR.idle)]
    ee_write -> page1 : {stat_wr = false}
    page4 -> ee_write3 [order 2] : [stat_wr && in(EEPROM_WR.idle)]
    ee_write3 -> page4 : {stat_wr = false}
    page3 -> ee_write2 [order 2] : [stat_wr && in(EEPROM_WR.idle)]
    ee_write2 -> page3 : {stat_wr = false}
    page5 -> ee_write4 [order 3] : [stat_wr && in(EEPROM_WR.idle)]
    ee_write4 -> page5 : {stat_wr = false}
    page6 -> ee_write5 [order 1] : [stat_wr && in(EEPROM_WR.idle)]
    ee_write5 -> page6 : {stat_wr = false}
  state EEPROM_WR [parallel]
    settings: executionOrder=1
    state idle
    state ee_idle
      % свободна ли EEPROM?
    state ee_wr
      ee_adr = adres_step
      ee_send = 0
      ee_send = uint16(Step_ret)
      % записываем в eeprom
    (default) -> EEPROM_WR.idle
    EEPROM_WR.idle -> ee_idle : ee_wr
    ee_wr -> EEPROM_WR.idle : [~ee_idle]% ждем окончания записи
        | {ee_en_wr = false}% отключаем запись eeprom
    ee_idle -> ee_wr : [~ee_idle && ~ee_en_rd && ~ee_en_wr]{ee_en_wr = true}
  state read_eeprom [parallel]
    settings: executionOrder=4
    state ee_idle1
    state ee_idle2
    state ee_rd
      % запускаем чтение с еепром
    state ready
      en: Step_ret = uint8(bitand(ee_read,255))
      ee_rd_ok = true
      ex: ee_en_rd = false % выключаем чтение из еепром
    state finish
    ee_idle2 -> ee_idle1 [order 2]
    (default) -> ee_idle1
    ee_idle1 -> ee_idle2 : [~ee_idl]
    ee_idle2 -> ee_rd [order 1] : [~ee_idl]{ee_adr = adres_step;ee_en_rd = true;}
    ee_rd -> ready : [~ee_idle] % дожидаемся конца чтения
    ready -> finish
  state buttons [parallel]
    settings: executionOrder=3
    state scan_buttons
    (default) -> scan_buttons
    scan_buttons -> (junction 284)
    (junction 284) -> (junction 287) [order 1] : [stepP && ~stats_in(1)]{stats_in(1) = true; step_P}
    (junction 287) -> (junction 289)
    (junction 284) -> (junction 289) [order 2]
    (junction 323) -> scan_buttons
    (junction 289) -> (junction 291) [order 1] : [~stepP && stats_in(1)]{stats_in(1) = false}
    (junction 291) -> (junction 294)
    (junction 289) -> (junction 294) [order 2]
    (junction 294) -> (junction 296) [order 1] : [stepM && ~stats_in(2)]{stats_in(2) = true; step_M}
    (junction 294) -> (junction 299) [order 2]
    (junction 299) -> (junction 301) [order 1] : [~stepM && stats_in(2)]{stats_in(2) = false}
    (junction 301) -> (junction 303)
    (junction 299) -> (junction 303) [order 2]
    (junction 303) -> (junction 323)
  state x = ee_idl [function]
    (default) -> (junction 169)
    (junction 169) -> (junction 170) [order 1] : [~ee_idle && ~ee_en_rd && ~ee_en_wr]
    (junction 170) -> (junction 172)
    (junction 169) -> (junction 171) [order 2] : {x=true}
    (junction 172) -> (junction 171) : {x = false}
  data: x function_output; adres_step constant uint8 =uint8(125); ee_idle data_store_memory; ee_adr data_store_memory; ee_en_rd data_store_memory; ee_read data_store_memory; ee_send data_store_memory; ee_en_wr data_store_memory; stat_wr local boolean size=1 =false; ee_rd_ok local boolean size=1 =false; stats_in local boolean size=[1 4] =false; Step_ret output uint8 size=1 =uint8(1); stepM input boolean size=1; stepP input boolean size=1
  events: ee_wr local FUNCTION_CALL_EVENT; step_P local RISING_EDGE_EVENT; step_M local RISING_EDGE_EVENT
